simulink model "attitudeEstimationVerification"  (R2018a)
settings: Solver=FixedStepAuto  StartTime=0.0  StopTime=120  FixedStep=0.001  RelTol=1e-3
undefined symbols (not defined in the file): SkywalkerX8
libraries: simulink_extras x8, sharedTrackingLibrary x1
settings Model: Creator=David  LastModifiedBy=David

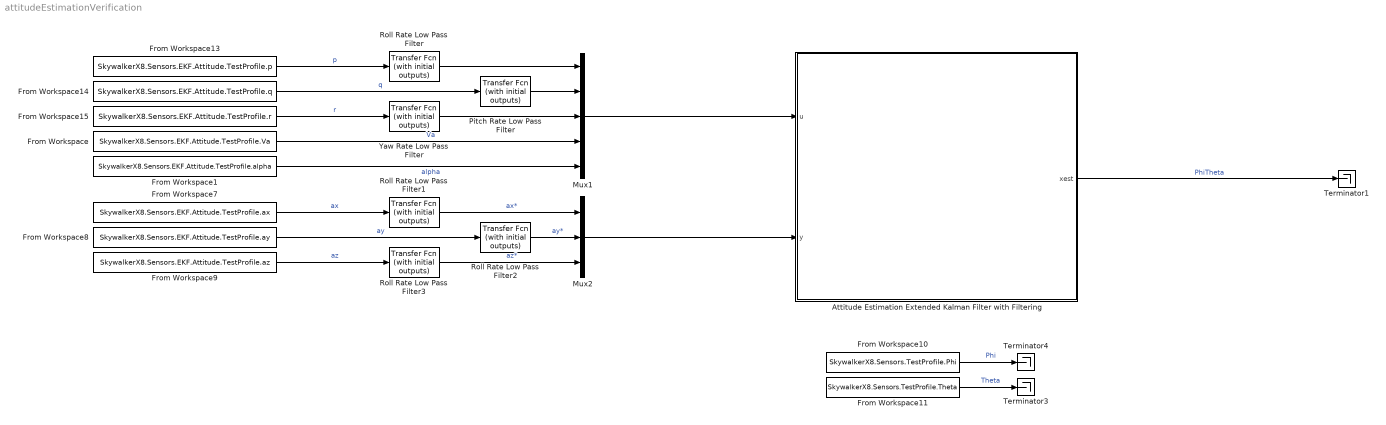
== system attitudeEstimationVerification ==
  Attitude Estimation Extended Kalman Filter with Filtering : Subsystem
      mask Display:
      | port_label('input', 1, '{\bf u} = [p, q, r, V_a, \alpha]', 'texMode', 'On')
      | port_label('input', 2, '{\bf y} = [a_x, a_y, a_z]', 'texMode', 'On')
      | 
      | port_label('output', 1, '{\bf x_{est}} = [\Phi, \theta]', 'texMode', 'On')
  From Workspace : FromWorkspace  VariableName=SkywalkerX8.Sensors.EKF.Attitude.TestProfile.Va  Interpolate=off  OutputAfterFinalValue=Holding final value
  From Workspace1 : FromWorkspace  VariableName=SkywalkerX8.Sensors.EKF.Attitude.TestProfile.alpha  Interpolate=off  OutputAfterFinalValue=Holding final value
  From Workspace10 : FromWorkspace  VariableName=SkywalkerX8.Sensors.TestProfile.Phi  Interpolate=off  OutputAfterFinalValue=Holding final value
  From Workspace11 : FromWorkspace  VariableName=SkywalkerX8.Sensors.TestProfile.Theta  Interpolate=off  OutputAfterFinalValue=Holding final value
  From Workspace13 : FromWorkspace  VariableName=SkywalkerX8.Sensors.EKF.Attitude.TestProfile.p  Interpolate=off  OutputAfterFinalValue=Holding final value
  From Workspace14 : FromWorkspace  VariableName=SkywalkerX8.Sensors.EKF.Attitude.TestProfile.q  Interpolate=off  OutputAfterFinalValue=Holding final value
  From Workspace15 : FromWorkspace  VariableName=SkywalkerX8.Sensors.EKF.Attitude.TestProfile.r  Interpolate=off  OutputAfterFinalValue=Holding final value
  From Workspace7 : FromWorkspace  VariableName=SkywalkerX8.Sensors.EKF.Attitude.TestProfile.ax  Interpolate=off  OutputAfterFinalValue=Holding final value
  From Workspace8 : FromWorkspace  VariableName=SkywalkerX8.Sensors.EKF.Attitude.TestProfile.ay  Interpolate=off  OutputAfterFinalValue=Holding final value
  From Workspace9 : FromWorkspace  VariableName=SkywalkerX8.Sensors.EKF.Attitude.TestProfile.az  Interpolate=off  OutputAfterFinalValue=Holding final value
  Mux1 : Mux  Inputs=5
  Mux2 : Mux  Inputs=3
  Pitch Rate Low Pass Filter : simulink_extras/Additional Linear/Transfer Fcn (with initial outputs)  N=cell2mat(SkywalkerX8.Sensors.Filters.AngularRates.Pitch.FilterTF.Numerator)  D=cell2mat(SkywalkerX8.Sensors.Filters.AngularRates.Pitch.FilterTF.Denominator)  Y0=SkywalkerX8.Sensors.Filters.AngularRates.Pitch.InitialCondition  U0=SkywalkerX8.Sensors.Filters.AngularRates.Pitch.InitialCondition
  Roll Rate Low Pass Filter : simulink_extras/Additional Linear/Transfer Fcn (with initial outputs)  N=cell2mat(SkywalkerX8.Sensors.Filters.AngularRates.Roll.FilterTF.Numerator)  D=cell2mat(SkywalkerX8.Sensors.Filters.AngularRates.Roll.FilterTF.Denominator)  Y0=SkywalkerX8.Sensors.Filters.AngularRates.Roll.InitialCondition  U0=SkywalkerX8.Sensors.Filters.AngularRates.Roll.InitialCondition
  Roll Rate Low Pass Filter1 : simulink_extras/Additional Linear/Transfer Fcn (with initial outputs)  N=cell2mat(SkywalkerX8.Sensors.EKF.Attitude.Filters.axFilterTF.Numerator)  D=cell2mat(SkywalkerX8.Sensors.EKF.Attitude.Filters.axFilterTF.Denominator)  Y0=SkywalkerX8.Sensors.EKF.Attitude.InitialMeasurement(1)  U0=SkywalkerX8.Sensors.EKF.Attitude.InitialMeasurement(1)
  Roll Rate Low Pass Filter2 : simulink_extras/Additional Linear/Transfer Fcn (with initial outputs)  N=cell2mat(SkywalkerX8.Sensors.EKF.Attitude.Filters.ayFilterTF.Numerator)  D=cell2mat(SkywalkerX8.Sensors.EKF.Attitude.Filters.ayFilterTF.Denominator)  Y0=SkywalkerX8.Sensors.EKF.Attitude.InitialMeasurement(2)  U0=SkywalkerX8.Sensors.EKF.Attitude.InitialMeasurement(2)
  Roll Rate Low Pass Filter3 : simulink_extras/Additional Linear/Transfer Fcn (with initial outputs)  N=cell2mat(SkywalkerX8.Sensors.EKF.Attitude.Filters.azFilterTF.Numerator)  D=cell2mat(SkywalkerX8.Sensors.EKF.Attitude.Filters.azFilterTF.Denominator)  Y0=SkywalkerX8.Sensors.EKF.Attitude.InitialMeasurement(3)  U0=SkywalkerX8.Sensors.EKF.Attitude.InitialMeasurement(3)
  Terminator1 : Terminator
  Terminator3 : Terminator
  Terminator4 : Terminator
  Yaw Rate Low Pass Filter : simulink_extras/Additional Linear/Transfer Fcn (with initial outputs)  N=cell2mat(SkywalkerX8.Sensors.Filters.AngularRates.Yaw.FilterTF.Numerator)  D=cell2mat(SkywalkerX8.Sensors.Filters.AngularRates.Yaw.FilterTF.Denominator)  Y0=SkywalkerX8.Sensors.Filters.AngularRates.Yaw.InitialCondition  U0=SkywalkerX8.Sensors.Filters.AngularRates.Yaw.InitialCondition
  wires:
  From Workspace8/1 -> Roll Rate Low Pass Filter2/1  "ay"
  From Workspace9/1 -> Roll Rate Low Pass Filter3/1  "az"
  From Workspace7/1 -> Roll Rate Low Pass Filter1/1  "ax"
  From Workspace/1 -> Mux1/4  "Va"
  From Workspace15/1 -> Yaw Rate Low Pass Filter/1  "r"
  From Workspace14/1 -> Pitch Rate Low Pass Filter/1  "q"
  From Workspace13/1 -> Roll Rate Low Pass Filter/1  "p"
  From Workspace11/1 -> Terminator3/1  "Theta"
  From Workspace10/1 -> Terminator4/1  "Phi"
  Roll Rate Low Pass Filter/1 -> Mux1/1
  Pitch Rate Low Pass Filter/1 -> Mux1/2
  Yaw Rate Low Pass Filter/1 -> Mux1/3
  Roll Rate Low Pass Filter1/1 -> Mux2/1  "ax*"
  Roll Rate Low Pass Filter2/1 -> Mux2/2  "ay*"
  Roll Rate Low Pass Filter3/1 -> Mux2/3  "az*"
  Mux1/1 -> Attitude Estimation Extended Kalman Filter with Filtering/1(u)
  Mux2/1 -> Attitude Estimation Extended Kalman Filter with Filtering/2(y)
  Attitude Estimation Extended Kalman Filter with Filtering/1(xest) -> Terminator1/1  "PhiTheta"
  From Workspace1/1 -> Mux1/5  "alpha"

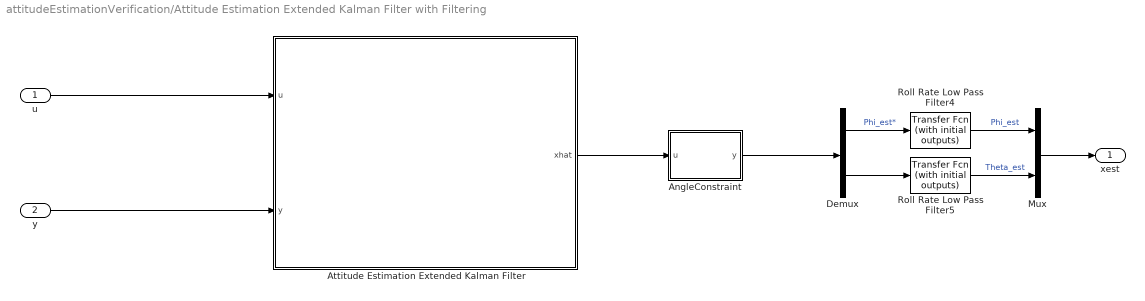
== system attitudeEstimationVerification/Attitude Estimation Extended Kalman Filter with Filtering ==
  u : Inport
  y : Inport  Port=2
  AngleConstraint : MATLAB Function  TreatAsAtomicUnit=on
  Attitude Estimation Extended Kalman Filter : Subsystem
      mask Display:
      | port_label('input', 1, '{\bf u} = [p, q, r, V_a, \alpha]', 'texMode', 'On')
      | port_label('input', 2, '{\bf y} = [a_x, a_y, a_z]', 'texMode', 'On')
      | 
      | port_label('output', 1, '{\bf x_{est}} = [\Phi, \theta]', 'texMode', 'On')
  Demux : Demux  Outputs=2
  Mux : Mux  Inputs=2
  Roll Rate Low Pass Filter4 : simulink_extras/Additional Linear/Transfer Fcn (with initial outputs)  N=cell2mat(SkywalkerX8.Sensors.EKF.Attitude.Filters.PhiFilterTF.Numerator)  D=cell2mat(SkywalkerX8.Sensors.EKF.Attitude.Filters.PhiFilterTF.Denominator)  Y0=SkywalkerX8.Sensors.EKF.Attitude.InitialState(1)  U0=SkywalkerX8.Sensors.EKF.Attitude.InitialState(1)
  Roll Rate Low Pass Filter5 : simulink_extras/Additional Linear/Transfer Fcn (with initial outputs)  N=cell2mat(SkywalkerX8.Sensors.EKF.Attitude.Filters.ThetaFilterTF.Numerator)  D=cell2mat(SkywalkerX8.Sensors.EKF.Attitude.Filters.ThetaFilterTF.Denominator)  Y0=SkywalkerX8.Sensors.EKF.Attitude.InitialState(2)  U0=SkywalkerX8.Sensors.EKF.Attitude.InitialState(2)
  xest : Outport
  wires:
  Demux/1 -> Roll Rate Low Pass Filter4/1  "Phi_est*"
  y/1 -> Attitude Estimation Extended Kalman Filter/2(y)
  Demux/2 -> Roll Rate Low Pass Filter5/1
  Roll Rate Low Pass Filter5/1 -> Mux/2  "Theta_est"
  AngleConstraint/1(y) -> Demux/1
  Attitude Estimation Extended Kalman Filter/1(xhat) -> AngleConstraint/1(u)
  Roll Rate Low Pass Filter4/1 -> Mux/1  "Phi_est"
  u/1 -> Attitude Estimation Extended Kalman Filter/1(u)
  Mux/1 -> xest/1

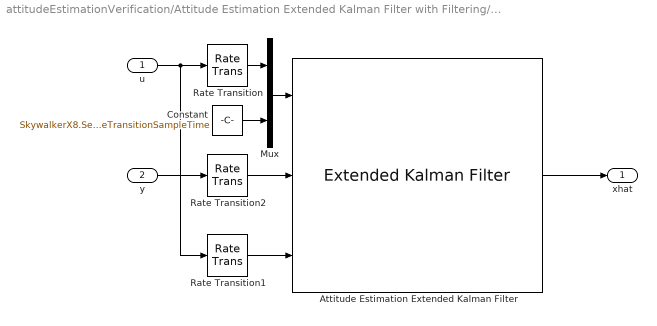
== system attitudeEstimationVerification/Attitude Estimation Extended Kalman Filter with Filtering/Attitude Estimation Extended Kalman Filter ==
  u : Inport
  y : Inport  Port=2
  Attitude Estimation Extended Kalman Filter : sharedTrackingLibrary/Extended Kalman Filter  StateTransitionFcn=attitudeTransitionEstimate  HasStateTransitionJacobianFcn=on  StateTransitionJacobianFcn=attitudeTransitionEstimate_Jacobian  HasAdditiveProcessNoise=Additive  ProcessNoise=SkywalkerX8.Sensors.EKF.Attitude.ProcessCovarianceMatrix  HasTimeVaryingProcessNoise=off  HasStateTransitionFcnExtraArgument=1  InitialState=SkywalkerX8.Sensors.EKF.Attitude.InitialState  InitialStateCovariance=SkywalkerX8.Sensors.EKF.Attitude.InitialStateCovarianceMatrix  MeasurementFcn1=accelerometerMeasurementEstimate  HasMeasurementJacobianFcn1=on  MeasurementJacobianFcn1=accelerometerMeasurementEstimate_Jacobian  HasMeasurementEnablePort1=off  HasAdditiveMeasurementNoise1=Additive  MeasurementNoise1=SkywalkerX8.Sensors.EKF.Attitude.MeasurementCovarianceMatrix  HasTimeVaryingMeasurementNoise1=off  HasMeasurementFcnExtraArgument1=1  MeasurementFcn2=myMeasurementFcn  HasMeasurementJacobianFcn2=off  HasMeasurementEnablePort2=off  HasAdditiveMeasurementNoise2=Additive  MeasurementNoise2=1  HasTimeVaryingMeasurementNoise2=off  HasMeasurementFcnExtraArgument2=0  MeasurementFcn3=myMeasurementFcn  HasMeasurementJacobianFcn3=off  HasMeasurementEnablePort3=off  HasAdditiveMeasurementNoise3=Additive  MeasurementNoise3=1  HasTimeVaryingMeasurementNoise3=off  HasMeasurementFcnExtraArgument3=0  MeasurementFcn4=myMeasurementFcn  HasMeasurementJacobianFcn4=off  HasMeasurementEnablePort4=off  HasAdditiveMeasurementNoise4=Additive  MeasurementNoise4=1  HasTimeVaryingMeasurementNoise4=off  HasMeasurementFcnExtraArgument4=0  MeasurementFcn5=myMeasurementFcn  HasMeasurementJacobianFcn5=off  HasMeasurementEnablePort5=off  HasAdditiveMeasurementNoise5=Additive  MeasurementNoise5=1  HasTimeVaryingMeasurementNoise5=off  HasMeasurementFcnExtraArgument5=0  EnableMultirate=on  StateTransitionFcnSampleTime=SkywalkerX8.Sensors.EKF.Attitude.StateTransitionSampleTime  MeasurementFcn1SampleTime=SkywalkerX8.Sensors.EKF.Attitude.MeasurementSampleTime  MeasurementFcn2SampleTime=1  MeasurementFcn3SampleTime=1  MeasurementFcn4SampleTime=1  MeasurementFcn5SampleTime=1  UseCurrentEstimator=on  OutputStateCovariance=off  DataType=double  SampleTime=SkywalkerX8.Sensors.EKF.Attitude.StateTransitionSampleTime  NumberOfMeasurements=1
      settings: SourceProductName=Control System Toolbox  SourceProductBaseCode=CT
  Constant : Constant  Value=SkywalkerX8.Sensors.EKF.Attitude.StateTransitionSampleTime
  Mux : Mux  Inputs=2
  Rate Transition : RateTransition  InitialCondition=SkywalkerX8.Sensors.EKF.Attitude.InitialInput  OutPortSampleTime=SkywalkerX8.Sensors.EKF.Attitude.StateTransitionSampleTime
  Rate Transition1 : RateTransition  InitialCondition=SkywalkerX8.Sensors.EKF.Attitude.InitialInput  OutPortSampleTime=SkywalkerX8.Sensors.EKF.Attitude.MeasurementSampleTime
  Rate Transition2 : RateTransition  InitialCondition=SkywalkerX8.Sensors.EKF.Attitude.InitialMeasurement  OutPortSampleTime=SkywalkerX8.Sensors.EKF.Attitude.MeasurementSampleTime
  xhat : Outport
  wires:
  y/1 -> Rate Transition2/1
  u/1 -> Rate Transition1/1, Rate Transition/1
  Attitude Estimation Extended Kalman Filter/1 -> xhat/1
  Rate Transition1/1 -> Attitude Estimation Extended Kalman Filter/3
  Rate Transition2/1 -> Attitude Estimation Extended Kalman Filter/2
  Mux/1 -> Attitude Estimation Extended Kalman Filter/1
  Rate Transition/1 -> Mux/1
  Constant/1 -> Mux/2

== matlab function attitudeEstimationVerification/Attitude Estimation Extended Kalman Filter with Filtering/AngleConstraint ==
  data: u input; y output
function y = fcn(u)

y = zeros(1, 2);

y(1) = asin(sin(u(1)));
y(2) = asin(sin(u(2)));
